simulink model "quatro_a"  (R2015a)
settings: Solver=ode45  StartTime=0.0  StopTime=10.0  RelTol=1e-3
settings Model: Creator=joao  LastModifiedBy=João F
settings DataIOCC: SignalLoggingSaveFormat=ModelDataLogs
settings OptimizationCC: ExpressionDepthLimit=2147483647
settings DebuggingCC: UnderspecifiedInitializationDetection=Classic  MergeDetectMultiDrivingBlocksExec=none  SolverPrmCheckMsg=warning  FcnCallInpInsideContextMsg=EnableAllAsWarning  StateNameClashWarn=warning
settings GRTTargetCC: CombineOutputUpdateFcns=off  GRTInterface=on

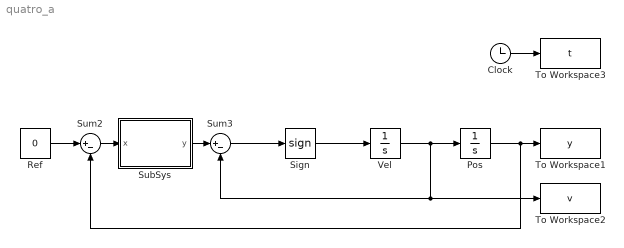
== system quatro_a ==
  Clock : Clock
  Pos : Integrator  InitialCondition=1
  Ref : Constant  Value=0
  Sign : Signum
  SubSys : MATLAB Function  TreatAsAtomicUnit=on
  Sum2 : Sum  Inputs=|+-
  Sum3 : Sum  Inputs=|+-
  To Workspace1 : ToWorkspace  VariableName=y  SampleTime=-1
  To Workspace2 : ToWorkspace  VariableName=v  SampleTime=-1
  To Workspace3 : ToWorkspace  VariableName=t  SampleTime=-1
  Vel : Integrator
  wires:
  Pos/1 -> Sum2/2, To Workspace1/1
  Vel/1 -> Pos/1, Sum3/2, To Workspace2/1
  Clock/1 -> To Workspace3/1
  Ref/1 -> Sum2/1
  Sum2/1 -> SubSys/1(x)
  SubSys/1(y) -> Sum3/1
  Sum3/1 -> Sign/1
  Sign/1 -> Vel/1

== matlab function quatro_a/SubSys ==
  data: x input; y output
function y = f(x)

y = sign(x)*sqrt(2*abs(x));
